simulink model "PIcf"  (R2016a)
settings: Solver=VariableStepAuto  StartTime=0.0  StopTime=20
libraries: fuzblock x1
settings Model: Creator=PC  LastModifiedBy=PC
settings SolverCC: ZeroCrossControl=DisableAll
settings DataIOCC: LimitDataPoints=on  SaveOutput=off  SaveTime=off  Refine=10
settings OptimizationCC: ExpressionDepthLimit=2147483647  LifeSpan=1
settings DebuggingCC: UnderspecifiedInitializationDetection=Classic  MergeDetectMultiDrivingBlocksExec=none  FcnCallInpInsideContextMsg=EnableAllAsWarning  AllowSymbolicDim=off  StateNameClashWarn=warning
settings GRTTargetCC: CombineOutputUpdateFcns=off  GRTInterface=on

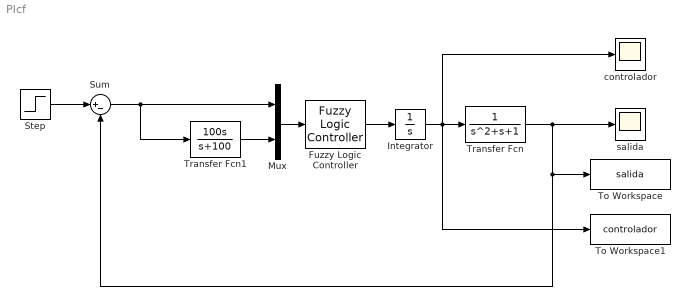
== system PIcf ==
  Fuzzy Logic Controller : fuzblock/Fuzzy Logic  Controller  fis=piDifuso
  Integrator : Integrator
  Mux : Mux  Inputs=2
  Step : Step  Time=0  SampleTime=0
  Sum : Sum  Inputs=|+-
  To Workspace : ToWorkspace  VariableName=salida  SaveFormat=Timeseries  SampleTime=-1
  To Workspace1 : ToWorkspace  VariableName=controlador  SaveFormat=Timeseries  SampleTime=-1
  Transfer Fcn : TransferFcn  Denominator=[1 1 1]
  Transfer Fcn1 : TransferFcn  Numerator=[100 0]  Denominator=[1 100]
  controlador : Scope
  "salida " : Scope
  wires:
  Step/1 -> Sum/1
  Transfer Fcn/1 -> "salida "/1, Sum/2, To Workspace/1
  Fuzzy Logic Controller/1 -> Integrator/1
  Mux/1 -> Fuzzy Logic Controller/1
  Sum/1 -> Mux/1, Transfer Fcn1/1
  Transfer Fcn1/1 -> Mux/2
  Integrator/1 -> controlador/1, Transfer Fcn/1, To Workspace1/1
